simulink model "sldemo_counters"  (Simulink 10.0)
settings: Solver=FixedStepDiscrete  StartTime=0.0  StopTime=2.25  FixedStep=.01  RelTol=1e-3  AbsTol=1e-6  EnableMultiTasking=on
Description:
  | Counters Using Conditionally Executed Subsystems
  | 
  | This model shows the contrast between enabled subsystems and triggered
  | subsystems for the same control signal, through the use of counter circuits.
  | After running the simulation, the scope shows three plots.
  | 
  | The first of these plots shows the control signal which is the output of the discrete
  | pulse generator.
  | 
  | The second plot shows the output of the counter circuit in the enabled subsystem.
  | The counter increments while the subsystem is enabled and then holds its output when
  | the subsystem is disabled. The counter resets to zero when the subsystem is re-enabled
  | because the enable port was configured to reset states when enabling.
  | 
  | The third plot shows the output of the counter circuit in the triggered subsystem. The
  | counter increments every rising edge of the control signal.
  | 
  | The signals are shown in a Signal Viewer scope that does not require a scope block to
  | be put into the block diagram.  Instead, the "scope" icon notation on the ports show
  | that a Signal Viewer is attached.  Double click on the scope icon to make the Signal
  | Viewer appear if it is hidden.
settings Model: Creator=The MathWorks, Inc.  LastModifiedBy=bhisma  ExtModeTrigMode=oneshot  ExtModeArmWhenConnect=off  ExtModeAutoUpdateStatusClock=off
settings SolverCC: AutoScaleAbsTol=off
settings DataIOCC: ReturnWorkspaceOutputs=on
settings OptimizationCC: BlockReduction=off  BooleanDataType=off  ExpressionDepthLimit=2147483647  InitFltsAndDblsToZero=on  BufferReusableBoundary=off
settings DebuggingCC: SaveWithParameterizedLinksMsg=none  SignalResolutionControl=TryResolveAllWithWarning  MultiTaskDSMMsg=warning  MultiTaskCondExecSysMsg=none  FcnCallInpInsideContextMsg=warning  BusObjectLabelMismatch=none  StateNameClashWarn=warning
settings HardwareCC: TargetUnknown=on
settings GRTTargetCC: TargetFcnLib=ansi_tfl_tmw.mat  GeneratePreprocessorConditionals=Disable all
settings ConfigComp: CovExternalEMLEnable=off  CovSFcnEnable=off

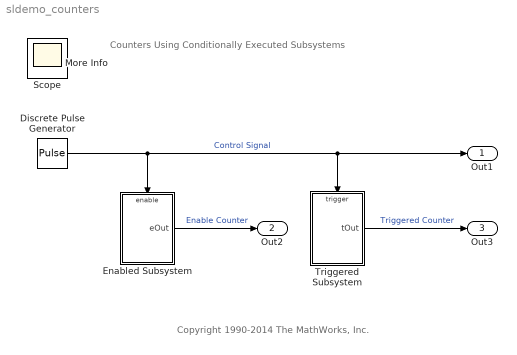
== system sldemo_counters ==
  note: Counters Using
      | Conditionally Executed Subsystems
  note: Copyright 1990-2014 The MathWorks, Inc.
  Discrete Pulse Generator : DiscretePulseGenerator  Period=40  PulseWidth=20  SampleTime=0.01
  Enabled Subsystem : Subsystem  TreatAsAtomicUnit=on
  More Info : Subsystem
      settings: OpenFcn=showExample('simulink_general/sldemo_countersExample')
      mask Display: disp('?')
  Triggered Subsystem : Subsystem  TreatAsAtomicUnit=on
  Out1 : Outport  VectorParamsAs1DForOutWhenUnconnected=off
  Out2 : Outport  Port=2  VectorParamsAs1DForOutWhenUnconnected=off
  Out3 : Outport  Port=3  VectorParamsAs1DForOutWhenUnconnected=off
  Scope : Scope
  wires:
  Discrete Pulse Generator/1 -> Enabled Subsystem/Enable, Triggered Subsystem/Trigger, Out1/1  "Control Signal"
  Triggered Subsystem/1(tOut) -> Out3/1  "Triggered Counter"
  Enabled Subsystem/1(eOut) -> Out2/1  "Enable Counter"

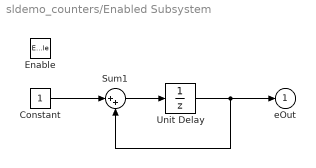
== system sldemo_counters/Enabled Subsystem ==
  Enable : EnablePort  StatesWhenEnabling=reset
  Constant : Constant
  Sum1 : Sum  Inputs=|++  SaturateOnIntegerOverflow=on  InputSameDT=on  OutDataTypeStr=Inherit: Same as first input
  Unit Delay : UnitDelay  SampleTime=.01  HasFrameUpgradeWarning=on
  eOut : Outport  InitialOutput=0  VectorParamsAs1DForOutWhenUnconnected=off
  wires:
  Sum1/1 -> Unit Delay/1
  Constant/1 -> Sum1/1
  Unit Delay/1 -> eOut/1, Sum1/2

== system sldemo_counters/More Info ==

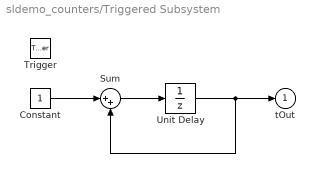
== system sldemo_counters/Triggered Subsystem ==
  Trigger : TriggerPort  VariantControl=Variant
  Constant : Constant
  Sum : Sum  Inputs=|++  SaturateOnIntegerOverflow=on  InputSameDT=on  OutDataTypeStr=Inherit: Same as first input
  Unit Delay : UnitDelay  SampleTime=-1  HasFrameUpgradeWarning=on
  tOut : Outport  InitialOutput=0  VectorParamsAs1DForOutWhenUnconnected=off
  wires:
  Sum/1 -> Unit Delay/1
  Constant/1 -> Sum/1
  Unit Delay/1 -> tOut/1, Sum/2
